simulink library "common_lib"  (R2021b)
settings: Solver=ode45  StartTime=0.0  StopTime=10.0  RelTol=1e-3
undefined symbols (not defined in the file or in its folder): ACCEL_PRE_MULT, C_C1GearNumbers, C_C1GearRatios, C_Calibration, C_DitherWaveform, C_GearOffset, C_GearRatioIn, C_GearRatioInverseOut, C_GearRatioOut, CLUTCH_INNER_LOOP_UPDATE_RATE, CONSTANT, DEGRADED_MODE_SIZE, Dem_EventStatusType, DiscIntNeverNeededParam, F_FAULT_ENUM, F_NOFAULT, F_OUTOFRANGE, F_RATELIMIT, FALSE, FMI14_SPECIAL_INSTRUCTIONS, FMI20_DATA_DRIFTED_HIGH, FMI21_DATA_DRIFTED_LOW, FMI29_RESERVED_FOR_SAE_ASSIGNMENT, FMI30_RESERVED_FOR_SAE_ASSIGNMENT, FMI31_CONDITION_EXISTS, FMI32_NO_FAULT, IC, k_accel, k_mean, LVDCU_OORH_FaultCntThd_C, MAX_UINT32, MEAN_PRE_MULT, NTriggers, QLTY_SIGNAL_FAILED, QLTY_SIGNAL_FULLY_FUNCTION, QLTY_SIGNAL_SUBSTITUTED_BY_1ST_CHOICE, QLTY_SIGNAL_SUBSTITUTED_BY_2ND_CHOICE, QLTY_SIGNAL_SUBSTITUTED_BY_3RD_CHOICE, QLTY_SIGNAL_SUBSTITUTED_BY_4TH_CHOICE, SAMPLE_TIME_100_mSec, SAMPLE_TIME_100_uSec, simin, T_TestPoint, TF_FALSE, TF_TRUE, TimeStep, TRUE, WORKSPACE_UPDATE_RATE, ZERO, Zero
libraries: $bdroot x120, simulink x27, simulink_extras x4, MBD_EPS_Local_Blockset x4
(part 2 of 10)

== system common_lib/Documentation ==
  note: Documentation
  EatonLogo : Subsystem
      mask Display: image('EatonLogo.jpg')
  LegalNoticeEaton : Subsystem  mask(LegalNotice){Company=Eaton Corporation}
      mask prompts: Company "Select Company"
      mask TypeOptions Company: Eaton Corporation | Eaton Cummins Automated Transmission Technologies
      mask Display:
      | corp = get_param(gcb,'Company');
      | disp(sprintf([...
      | 'Unpublished Work\n',...
      | 'Copyright %s %s.\n',...
      | 'Notice:\n',...
      | 'This document contains confidential information.\n',...
      | 'Disclosure of this information is conditioned upon the recipient''s agreement that\n',...
      | 'the use of the information shall be only for the purpose motivating the disclosure.\n',...
      | 'Any other use is strictly prohibited without the prior written consent.'],...
      | datestr(now,'yyyy'),corp))
  RequirementLinks : Subsystem  mask(ReqLink){}
      settings: OpenFcn=open_system([gcb '/DocBlock'])
      mask Display:
      | a = get_param([gcb '/DocBlock'],'UserData');
      | if isempty(a)
      |     disp('Double Click to Open');
      | else
      |     disp(sprintf('Requirements (REQ_####)\n%s',a.content));
      | end
  SubsystemPath : Subsystem  mask(SubSysPathInfo){}
      mask Display: disp(regexprep(get_param(gcb,'parent'),'/','>'))

== system common_lib/Fltrs ==
  note: Filters
  Fltr : Subsystem  RTWFcnName=FLTR  mask(CL Filter){TimeStep=[]}
      mask prompts: TimeStep "Time Step"
      mask help:
      | First Order Filter, y(n)= T/tau x(n) + (1 - T/tau) y(n-1)
      |
      | output = previous output + (input - previous output) * T/tau
      |
      | X(1) = input
      | X(2) = tau
      |
      | Y(1) = output
      |
      | Time step is entered via mask parameter.
      | NgEK, Inc.
      mask init:
      | %switch class(TimeStep)
      | %   case ('double')
      | %      IC = double(0.0);
      | %   case ('single')
      |        IC = single(0.0);
      | %   case ('int8')
      | %      IC = int8(0);
      | %   case ('int16')
      | %      IC = int16(0);
      | %   case ('int32')
      | %      IC = int32(0);
      | %end;
      | Ts = single(TimeStep);
      settings: RTWFcnNameOpts=User specified  RTWFileNameOpts=Use function name
      mask Help: web(which(['common_lib16.html']))
      mask Display:
      | patch([0.35 0.35 0.65 0.65], [0.4 0.6 0.6 0.4], [255/255 127/255 255/255])
      | disp('Filter')
      | port_label('input', 1, 'input')
      | port_label('input', 2, 'tau')
      | port_label('output', 1, 'output')
  Fltr_wR : Subsystem  mask(CL Filter wRO){TimeStep=[]}
      mask prompts: TimeStep "Time Step"
      mask help:
      | First Order Filter, y(n)= T/tau x(n) + (1 - T/tau) y(n-1)
      |
      | If      reset is true (1) then output=initial condition
      |    otherwise output = previous output + (input - previous output) * T/tau
      |
      | X(1) = input
      | X(2) = tau
      | X(3) = initial condition
      | X(4) = reset flag
      |
      | Y(1) = output
      |
      | Time step is entered via mask parameter.
      | NgEK, Inc.
      mask init: same as common_lib/Fltrs/Fltr
      mask Help: web(which(['common_lib18.html']))
      mask Display:
      | patch([0.4 0.4 0.6 0.6], [0.35 0.65 0.65 0.35], [255/255 127/255 255/255])
      | disp('Filter\nw R')
      | port_label('input', 1, 'input')
      | port_label('input', 2, 'tau')
      | port_label('input', 3, 'ic')
      | port_label('input', 4, 'reset?')
      | port_label('output', 1, 'output')
  Fltr_wRO : Subsystem  RTWFcnName=FLTRWRO  mask(CL Filter wRO){TimeStep=[]}
      mask prompts: TimeStep "Time Step"
      mask help:
      | First Order Filter, y(n)= T/tau x(n) + (1 - T/tau) y(n-1)
      |
      | If override is true (1) then output=override_value
      | If      reset is true (1) then output=input
      |    otherwise output = previous output + (input - previous output) * T/tau
      |
      | X(1) = input
      | X(2) = tau
      | X(3) = override value
      | X(4) = override flag
      | X(5) = reset flag
      |
      | Y(1) = output
      |
      | Time step is entered via mask parameter.
      | NgEK, Inc.
      mask init:
      | %switch class(TimeStep)
      | % case ('double')
      | %      IC = double(0.0);
      | %    case ('single')
      |        IC = single(0.0);
      | %    case ('int8')
      | %         IC = int8(0);
      | %    case ('int16')
      | %      IC = int16(0);
      | %   case ('int32')
      | %        IC = int32(0);
      | %end;
      | Ts = single(TimeStep);
      settings: RTWFcnNameOpts=User specified  RTWFileNameOpts=Use function name
      mask Help: web(which(['common_lib17.html']))
      mask Display:
      | patch([0.4 0.4 0.6 0.6], [0.35 0.65 0.65 0.35], [255/255 127/255 255/255])
      | disp('Filter\nw RO')
      | port_label('input', 1, 'input')
      | port_label('input', 2, 'tau')
      | port_label('input', 3, 'override_value')
      | port_label('input', 4, 'override?')
      | port_label('input', 5, 'reset?')
      | port_label('output', 1, 'output')
  Fltr_wROExtInitCond : Subsystem  TreatAsAtomicUnit=on  RTWFcnName=FLTRWRO  mask(CL Filter wRO wIC){TimeStep=[]}
      mask prompts: TimeStep "Time Step"
      mask help:
      | First Order Filter, y(n)= T/tau x(n) + (1 - T/tau) y(n-1)
      |
      | If override is true (1) then output=override_value
      | If      reset is true (1) then output=input
      |    otherwise output = previous output + (input - previous output) * T/tau
      |
      | X(1) = input
      | X(2) = tau
      | X(3) = inititial condition
      | X(4) = reset
      | X(5) = override TO
      | X(6) = override value TC
      | Y(1) = output
      mask init:
      | %switch class(TimeStep)
      | % case ('double')
      | %      IC = double(0.0);
      | %    case ('single')
      | %       IC = single(0.0);
      | %    case ('int8')
      | %         IC = int8(0);
      | %    case ('int16')
      | %      IC = int16(0);
      | %   case ('int32')
      | %        IC = int32(0);
      | %end;
      | %task_rate = single(taskrate_input);
      | Ts = single(TimeStep);
      settings: RTWFcnNameOpts=User specified  RTWFileNameOpts=Use function name
      mask Help: web(which(['common_lib17.html']))
      mask Display:
      | patch([0.2 0.2 0.8 0.8], [0.35 0.65 0.65 0.35], [255/255 127/255 255/255])
      | disp('Filter\n w ROExtInitCond')
      | port_label('input', 1, 'input')
      | port_label('input', 2, 'tau')
      | port_label('input', 3, 'ic')
      | port_label('input', 4, 'reset?')
      | port_label('input', 5, 'override?')
      | port_label('input', 6, 'override_value')
      | port_label('output',1, 'output')
  Int16FIR : Subsystem  mask(FIRInt16){N=50, Ts=0.01}
      mask prompts: N "Half Window Size (samples)"; Ts "Time Step"
      mask help:
      | Highly optimized FIR filter designed to calculated mean and least squares fit slope.
      |
      | For best results scale the input to use the whole range of int16, but note acceleration can saturate.  The buffer initializes to zero.
      |
      | Termination of an output will eliminate relevant code to calculate that output.
      mask init:
      | [k_mean, MEAN_PRE_MULT, k_accel, ACCEL_PRE_MULT] = FixedPointFIRInit(N,Ts);
      mask Display:
      | patch([0.35 0.35 0.65 0.65], [0.4 0.6 0.6 0.4], [255/255 127/255 255/255])
      | disp('Int16 FIR')
      | port_label('input', 1, 'u')
      | port_label('output', 1, 'mean')
      | port_label('output', 2, 'accel')
  Inv_Fltr : Subsystem  mask(CL Inverse Filter){TimeStep=[]}
      mask prompts: TimeStep "Time Step"
      mask help:
      | Inverse First Order Filter
      | u(k) = y(k-1) + tau/TimeStep*(y(k) - y(k-1))
      |
      | X(1) = input
      | X(2) = tau
      |
      | Y(1) = output
      |
      | Time step is entered via mask parameter.
      | NgEK, Inc.
      mask init:
      | %switch class(TimeStep)
      | %   case ('double')
      | %      Zero = double(0.0);
      | %   case ('single')
      |        Zero = single(0.0);
      | %   case ('int8')
      | %      Zero = int8(0);
      | %   case ('int16')
      | %      Zero = int16(0);
      | %   case ('int32')
      | %      Zero = int32(0);
      | %end;
      mask Help: web(which(['common_lib47.html']))
      mask Display:
      | patch([0.35 0.35 0.65 0.65], [0.3 0.7 0.7 0.3], [255/255 127/255 255/255])
      | disp('Inverse\nFilter')
      | port_label('input', 1, 'input')
      | port_label('input', 2, 'tau')
      | port_label('output', 1, 'output')
  Inv_RpdFltr : Subsystem  mask(CL Inverse Rapid Filtering){DType=Single}
      mask prompts: DType "Data Type"
      mask help:
      | Inverse of the Rapid Filter.  u(k) = y(k-1) + (y(k) - y(k-1))/fc
      |
      | X(1) = input
      | X(2) = filter constant
      |
      | Y(1) = output
      | NgEK, Inc.
      mask init:
      | switch class(TimeStep)
      |     case ('double')
      |         Zero = double(0.0);
      |     case ('single')
      |         Zero = single(0.0);
      |     case ('int8')
      |         Zero = int8(0);
      |     case ('int16')
      |         Zero = int16(0);
      |     case ('int32')
      |         Zero = int32(0);
      | end;
      mask Help: web(which(['common_lib48.html']))
      mask TypeOptions DType: Double | Single | Int8 | Int16 | Int32
      mask Display:
      | patch([0.30 0.30 0.70 0.70], [0.25 0.75 0.75 0.25], [255/255 127/255 255/255])
      | disp('Inverse\nRapid\nFiltering')
      | port_label('input', 1, 'input')
      | port_label('input', 2, 'fltr_cnst')
      | port_label('output', 1, 'output')
  Lookup_wFltr : Subsystem  mask(CL Filter wRO wIC wLut){TimeStep=[], Mode=Linear Interpolation}
      mask prompts: TimeStep "Time Step"; Mode "Interpolation Mode"
      mask help:
      | This block combines a 2D Table lookup with explicit axis inputs with a First Order Filter.
      |
      | First Order Filter, y(n)= T/tau x(n) + (1 - T/tau) y(n-1)
      |
      | If override is true (1) then output=override_value
      | If reset is true (1) then output=lookup_table_interpolation
      |    otherwise output = previous output + (lookup_table_interpolation - previous output) * T/tau
      |
      | X(1) = Independent variable
      | X(2) = X axis vector
      | X(3) = Y axis vector
      | X(4) = Override TO
      | X(5) = Override value TC
      | X(6) = Filter enable
      | X(7) = Filter tau
      | X(8) = Filter initial condition
      | Y(1) = Output
      |
      | Interpolation mode is selected via the mask:
      |
      | Ceiling Interpolation: rounds up in the positive direction
      | Floor Interpolation: rounds down in the negative direction
      | Nearest (Neighbor) Interpolation: rounds to the closest representable number
      | Linear Interpolation: Interpolates data by assuming data varies linearly between points
      mask init: same as common_lib/Fltrs/Fltr_wROExtInitCond
      mask TypeOptions Mode: Linear Interpolation | Nearest Neighbor | Floor | Ceiling
      mask Display:
      | patch([0.30 0.30 0.70 0.70], [0.45 0.55 0.55 0.45], [255/255 127/255 255/255])
      | disp('Lookup_wFltr')
      | port_label('input', 1, 'input')
      | port_label('input', 2, 'x-axis vector')
      | port_label('input', 3, 'y-axis vector' )
      | port_label('input', 4, 'override?')
      | port_label('input', 5, 'override_value')
      | port_label('input', 6, 'filter_enable?')
      | port_label('input', 7, 'tau')
      | port_label('input', 8, 'ic')
      | port_label('output', 1, 'output')
  Rpd_Fltr : Subsystem  mask(CL Rapid Filter){DType=Single}
      mask prompts: DType "Data Type"
      mask help:
      | Rapid 1st Order Filter, y(k)=x(k) + Fc*( Y(k-1) - X(k) )
      |
      | X(1) = input
      | X(2) = filter constant
      |
      | Y(1) = output
      | NgEK, Inc.
      mask init:
      | switch DType
      |    case (1)
      |        IC = double(0.0);
      |   case (2)
      |        IC = single(0.0);
      |    case (3)
      |          IC = int8(0);
      |     case (4)
      |          IC = int16(0);
      |    case (5)
      |        IC = int32(0);
      | end;
      mask Help: web(which(['common_lib19.html']))
      mask TypeOptions DType: Double | Single | Int8 | Int16 | Int32
      mask Display:
      | patch([0.35 0.35 0.65 0.65], [0.35 0.65 0.65 0.35], [255/255 127/255 255/255])
      | disp('Rapid\nFilter')
      | port_label('input', 1, 'input')
      | port_label('input', 2, 'fltr_cnst')
      | port_label('output', 1, 'output')
  Scaling_wFltr : Subsystem  mask(CL Filter wRO wIC wScl){TimeStep=[]}
      mask prompts: TimeStep "Time Step"
      mask help:
      | This block adds sclaing to scale the raw input signal. The signal is then filtered using first order filter.
      |
      | First Order Filter, y(n)= T/tau x(n) + (1 - T/tau) y(n-1)
      |
      | If override is true (1) then output=override_value
      | If reset is true (1) then output=input*resolution+offset
      |    otherwise output = previous output + ((input*resolution+offset) - previous output) * T/tau
      |
      | X(1) = input
      | X(2) = resolution
      | X(3) = offset
      | X(4) = override TO
      | X(5) = override value TC
      | X(6) = filter enable
      | X(7) = filter tau
      | X(8) = filter initial condition
      | Y(1) = output
      mask init: same as common_lib/Fltrs/Fltr_wROExtInitCond
      mask Display:
      | patch([0.30 0.30 0.70 0.70], [0.45 0.55 0.55 0.45], [255/255 127/255 255/255])
      | disp('Scaling_wFltr')
      | port_label('input', 1, 'input')
      | port_label('input', 2, 'res')
      | port_label('input', 3, 'offset' )
      | port_label('input', 4, 'override?')
      | port_label('input', 5, 'override_value')
      | port_label('input', 6, 'filter_enable?')
      | port_label('input', 7, 'tau')
      | port_label('input', 8, 'ic')
      | port_label('output', 1, 'output')

== system common_lib/Fuzzy ==
  note: Fuzzy Controller Design
  Demux : Demux  Outputs=2
  Fuzzy Implication : Subsystem  mask(CL Fuzzy Implication){from=ShiftPoint, value=HighUpshiftPoint}
      mask prompts: from "Result Bus Goto Tag"
      mask help:
      | The fuzzy implication is the final result of a decision tree branch.
      |
      | The value parameter of this block selects from the Result Bus the particular value that the output should take on when the associated branch is true.
      |
      | It is ok and likely to have multiple branches that result in the same value.  Adding all the result branches together will give a weight sum of the result.
      mask init:
      | set_param([gcb '/From'],'GotoTag',get_param(gcb,'from'));
      | set_param([gcb '/Select'],'OutputSignals',get_param(gcb,'value'))
      mask Display:
      | patch([0.25 0.25 0.75 0.75], [0.25 0.75 0.75 0.25], [255/255 127/255 255/255])
      | port_label('input',1,'THEN');
      | disp([get_param(gcb,'from') ' is\n' get_param(gcb,'value')])
  Fuzzy Intersection : Subsystem  mask(CL Fuzzy Decision){from=DataBus, signal=Demand, value=value, dispStr=Demand is\nvalue}
      mask prompts: from "Data Bus Goto Tag"; signal "Signal Name"; value "Value(s) (Comma seperated list of named values)"
      mask help:
      | The Fuzzy Decision block serves as the fuzzy AND operator.
      |
      | Input - Truth of previous statements.
      | TRUE Output - Incoming truth AND truth of selected signal values(s).
      | FALSE Output - Incoming truth AND falseness of selected signal values(s).
      |
      | TRUE Output + FALSE Output = Input
      mask init:
      | fromDlg = get_param(gcb,'from');
      | fromBlk = get_param([gcb '/From'],'GotoTag');
      | if ~strcmp(fromDlg,fromBlk)
      |    set_param([gcb '/From'],'GotoTag',get_param(gcb,'from'));
      | end
      | 
      | remain = strtrim(get_param(gcb,'value'));
      | first = true;
      | output = '';
      | sig = get_param(gcb,'signal');
      | dstr = [sig ' is\n'];
      | while any(remain)
      |     [str, remain] = strtok(remain,{',',' '});
      |     if first
      |         output = [sig '.' str];
      |         dstr = [dstr str];
      |     else
      |         output = [output ',' sig '.' str];
      |         dstr = [dstr '\nOR ' str];
      |     end
      |     first = false;
      | end
      | 
      | if ~strcmp(get_param(gcb,'dispStr'),dstr) || ...
      |    ~strcmp(get_param([gcb '/Select'],'OutputSignals'),output)
      |    set_param(gcb,'dispStr',dstr);
      | 
      |    %Delete old lines
      |    sel = get_param([gcb '/Select'],'PortHandles');
      |    n = length(sel.Outport);
      |    for i = 1:n
      |        line = get(sel.Outport(i),'Line');
      |        if line>0
      |            delete_line(line);
      |        end
      |    end
      | 
      |    %Set the new outputs
      |    set_param([gcb '/Select'],'OutputSignals',output)
      | 
      |    %Add new lines
      |    sel = get_param([gcb '/Select'],'PortHandles');
      |    n = length(sel.Outport);
      |    set_param([gcb '/OR'],'Inputs',char(ones(1,n)*'+'));
      |    for i = 1:n
      |        istr = num2str(i);
      |        add_line(gcb,['Select/' istr],['OR/' istr]);
      |    end
      | end
      mask Help:
      | The Fuzzy Decision block serves as the fuzzy AND operator.  The TRUE output
      | is the truth of the input AND truth of the selected signal value(s).  The
      | FALSE output is truth of the input but falseness of the selected signal
      | value(s).  Thus the sum of TRUE and FALSE output will equal the truth of
      | the input.
      | 
      | Use this block as nodes in a binary decision tree.  The root node should
      | always have an input truth of 1.0, the sum of all branches.  At the end of
      | each branch should be a Fuzzy THEN statement followed by a summation of all
      | THEN statements.
      mask Callback value:
      | if isempty(strtrim(get_param(gcb,'value')))
      |     set_param(gcb,'value','value');
      | end
      mask Display:
      | patch([0.25 0.25 0.75 0.75], [0.25 0.75 0.75 0.25], [255/255 127/255 255/255])
      | port_label('input',1,'IF');
      | port_label('output',1,'THEN');
      | port_label('output',2,'ELSE');
      | disp(get_param(gcb,'dispStr'))
  Fuzzy Membership Function : Subsystem  mask(CL Fuzzy Membership){}
      mask help:
      | This fuzzy membership function uses triangular functions centered at the breakpoints defined by the second input.  A ramp function is used for the first and last break point.
      |
      | This membership function enforces the property of mutual exclusivity.  The sum of all memberships equals 1.0 for the range of the input.
      |
      | The breakpoints must be in increasing order and be unique.  If not, order and uniqueness will be enforced by shifting breakpoints above the previously listed value in an iterative fasion.
      |
      | First Input - Input signal
      | Second Input - Breakpoint list
      mask Display:
      | patch([0.22 0.22 0.8 0.8], [0.3 0.68 0.68 0.3], [255/255 127/255 255/255])
      | plot([0.0 0.4 0.4],[0.8 0.8 0.7]);
      | text(0.15,0.65,'1');
      | plot([0.2 0.3 0.5 0.8],[0.7 0.7 0.3 0.3]);
      | plot([0.3 0.5 0.7],[0.3 0.7 0.3]);
      | text(0.15,0.35,'0');
      | plot([0.2 0.5 0.7 0.8],[0.3 0.3 0.7 0.7]);
      | 
      | 
      | plot([0.0 0.3 0.3 0.3 0.5 0.5 0.5 0.7 0.7],[0.2 0.2 0.25 0.2 0.2 0.25 0.2 0.2 0.25])
  Fuzzy Union : Sum  Inputs=|++
  Goto Tag Visibility : GotoTagVisibility  GotoTag=DataBus
  Goto Tag Visibility1 : GotoTagVisibility  GotoTag=ResultBus
  Truth : Constant  Value=single(1.0)  SampleTime=-1

== system common_lib/Gear Ratios ==
  note: Gear Ratios
  FindGearNumberByRatio : Subsystem  mask{RatioToGearIn=C_C1GearRatios, RatioToGearOut=C_C1GearNumbers, GearToRatioIn=C_GearRatioIn, GearToRatioOut=C_GearRatioOut, ConfirmTime=single(0), TimeStep=0.001}
      mask prompts: RatioToGearIn "RatioToGearIn (single)"; RatioToGearOut "RatioToGearOut (single)"; GearToRatioIn "GearToRatioIn (single)"; GearToRatioOut "GearToRatioOut (single)"; ConfirmTime "Speeed Confirmation Time (single)"; TimeStep "Time Step (double)"
      mask help:
      | This block outputs the GearNumber closest to the ratio appearing at the
      | input.  The block requires monotonically increasing tables.  i.e. the
      | RatioToGearIn and GearToRatioIn values must be increasing.
      |
      | The block works for both forward and reverse ratios.  (Positive and negative
      | speed and ratio).
      |
      | GearNumber - The gear number of the determined ratio.  Set to single(0) if
      | ratio does not match an available ratio.
      |
      | OutputValid - True if the ratio matches for ConfirmTime and above MinSpeed.
      |
      | SpeedAboveMin - True if speed is above MinSpeed.
      |
      | Ratio = ClutchSpeed/OutputSpeed
  GearNumberToRatio : Subsystem
      mask Display:
      | patch([0.3 0.3 0.7 0.7], [0.4 0.6 0.6 0.4], [255/255 127/255 255/255]);
      | disp('Gear Num\n to Ratio')
      | port_label('input',1,'gear_num')
      | port_label('output',1,'ratio')
      | port_label('output',2,'inv_ratio')

== system common_lib/IO ==
  note: IO Blocks
  Calibration with Pretty Print Value : Subsystem  mask(Calibratible Input){CalValue=C_Calibration, scaling=None}
      mask prompts: CalValue "Calibratible Name"
      mask help:
      | This block is simply a standard Simulink constant block w/ a custom wrapper to pretty-print the calibratible value on the mask.
      |
      | NgEK, Inc.
      mask init:
      | CalName = get_param(gcb,'CalValue');
      mask TypeOptions scaling: None | RPM | MPH
      mask Display:
      | fprintf([CalName ' = ' num2str(double(CalValue)*...
      |     (strcmp(get_param(gcb,'scaling'),'RPM')*30/pi+...
      |      strcmp(get_param(gcb,'scaling'),'MPH')*2.236936292+...
      |      strcmp(get_param(gcb,'scaling'),'None')*1.0)) ' '...
      |      char(strcmp(get_param(gcb,'scaling'),'RPM')*double('RPM')+...
      |           strcmp(get_param(gcb,'scaling'),'MPH')*double('MPH')+...
      |           strcmp(get_param(gcb,'scaling'),'None')*double(sprintf('   ')))])
  Calibration with Pretty Print Value1 : $bdroot/IO/Calibration with Pretty Print Value  CalValue=c_Calibration  scaling=None
  From Workspace w/Datatype : Subsystem  mask(From Workspace w/Datatype){st=0, var=simin, intdat=on, zerocross=off, extmode=Extrapolation}
      mask prompts: st "sample time"; var "data"; intdat "Interpolate data"; zerocross "Enable zero crossing detection"; extmode "Form output after final data value by:"
      mask help:
      | From worspace block with data type convertor at its output.
      |
      | NgEK, Inc.
      mask init:
      | dt = get_param(gcb,'st');
      | data = get_param(gcb,'var');
      | blk = [gcb '/From' sprintf('\n') 'Workspace'];
      | if intdat, mode = 'on'; else mode = 'off'; end
      | set_param(blk,'interpolate',mode)
      | if zerocross, mode = 'on'; else mode = 'off'; end
      | set_param(blk,'zerocross',mode)
      | switch extmode
      |     case 1
      |         mode = 'Extrapolation';
      |     case 2
      |         mode = 'Setting to zero';
      |     case 3
      |         mode = 'Hold final value';
      |     case 4
      |         mode = 'Cyclic repetition';
      | end
      | set_param(blk,'outputafterfinalvalue',mode)
      mask Help: Use just like the original from workspace block.
      mask TypeOptions extmode: Extrapolation | Setting to zero | Holding final value | Cyclic repetition
      mask Display: disp(data)
  Triangle : Subsystem  mask(CL Triangle){TimeStep=[]}
      mask prompts: TimeStep "Time Step"
      mask help:
      | Output a triangle signal of specified amplitude, offset and frequency.
      |
      | X(1) = amplitude
      | X(2) = frequency
      | X(3) = offset
      |
      | Y(1) = output
      |
      | Time step is entered via mask parameter.
      | NgEK, Inc.
      mask init:
      | h=[gcb '/Data Type Conversion'];
      | 
      | %switch class(TimeStep)
      | %   case ('double')
      | %      Zero        = double( 0.0);
      | %      ZeroZeroOne = double( 0.001);
      | %      One         = double( 1.0);
      | %      Two         = double( 2.0);
      | %      MinusOne    = double(-1.0);
      | %      set_param(h, 'DataType','double');
      | %      set_param([h '1'], 'DataType','double');
      | %   case ('single')
      |        Zero        = single( 0.0);
      |        ZeroZeroOne = single( 0.001);
      |        One         = single( 1.0);
      |        Two         = single( 2.0);
      |        MinusOne    = single(-1.0);
      |        set_param(h, 'DataType','single');
      |        set_param([h '1'], 'DataType','single');
      | %end;
      mask Help: web(which(['common_lib20.html']))
      mask Display:
      | patch([0.375 0.375 0.625 0.625], [0.35 0.65 0.65 0.35], [255/255 127/255 255/255])
      | plot([0.375 0.4375 .5 0.5625 0.625],[0.35 0.65 0.35 0.65 0.35]);
      | port_label('input', 1, 'amplitude')
      | port_label('input', 2, 'frequency')
      | port_label('input', 3, 'offset')
      | port_label('output', 1, 'output')

== system common_lib/Integrators ==
  note: Integrators
  ForwardEulerIntergrator : Subsystem  mask{IC=0, TSAMP=0}
      mask prompts: IC "Initial Condition"; TSAMP "Sample Time"
      mask Display:
      | patch([0.35 0.35 0.65 0.65], [0.3 0.7 0.7 0.3], [255/255 127/255 255/255])
      | disp('Forward Euler\nIntegral')
      | port_label('input',1,'dx')
      | port_label('input',2,'x0')
      | port_label('input',3,'reset')
      | port_label('output',1,'x')

== system common_lib/Misc ==
  note: Miscellaneous Computations
  ArcSine : Subsystem  mask(CL Trigonometric Function ArcSine){}
      mask help:
      | Simple trigonometric arcsine function.  The sine is the input and the angle is the output.
      |
      | This block is single precision.  The calculation used to determine arcsine is dervied from a Taylor Series approximation.  Note there are limitations with this approximation such as round off error.
      |
      | NgEK, Inc.
      mask Help: web(which(['common_lib51.html']))
      mask Display:
      | patch([0.30 0.30 0.70 0.70], [0.25 0.75 0.75 0.25], [255/255 127/255 255/255])
      | plot(linspace(-1,1,20)/6+0.5,(asin(linspace(-1,1,20)))/6.28+0.5)
  ClampAboveZero : Subsystem  mask(CL Clamp Above Zero){Tol=[]}
      mask prompts: Tol "Tolerance"
      mask help:
      | Clamps input above zero according to a calibratible tolerance.
      |
      | X(1) = input
      |
      | Y(1) = output
      | NgEK, Inc.
      settings: AttributesFormatString=tol=%<Tol>
      mask Help: web(which(['common_lib21.html']))
      mask Display:
      | patch([0.3 0.3 0.7 0.7], [0.35 0.65 0.65 0.35], [255/255 127/255 255/255])
      | 
      | plot([0 1],[0.5 0.5], [0.5 0.5],[0 1], [0 0.5 1], [0.55 0.55 1])
  ClampAroundZero : Subsystem  mask(CL Clamp Around Zero){Tol=[]}
      mask prompts: Tol "Tolerance"
      mask help:
      | Clamps input around zero according to a calibratible tolerance.
      |
      | X(1) = input
      |
      | Y(1) = output
      | NgEK, Inc
      mask init:
      | switch class(Tol)
      |   case ('double')
      |       One      = double(1.0);
      |        Zero     = double(0.0);
      |        MinusOne = double(-1.0);
      |  case ('single')
      |         One      = single(1.0);
      |        Zero     = single(0.0);
      |          MinusOne = single(-1.0);
      |  case ('int8')
      |         One      = int8(1.0);
      |          Zero     = int8(0.0);
      |          MinusOne = int8(-1.0);
      |     case ('int16')
      |        One      = int16(1.0);
      |         Zero     = int16(0.0);
      |         MinusOne = int16(-1.0);
      |   case ('int32')
      |         One      = int32(1.0);
      |         Zero     = int32(0.0);
      |         MinusOne = int32(-1.0);
      | end;
      settings: AttributesFormatString=tol=%<Tol>
      mask Help: web(which(['common_lib22.html']))
      mask Display:
      | patch([0.3 0.3 0.7 0.7], [0.35 0.65 0.65 0.35], [255/255 127/255 255/255])
      | 
      | plot([0 1],[0.5 0.5], [0.5 0.5],[0 1], [0 0.3 0.5 0.5 0.7 1], [0 0.3 0.3 0.7 0.7 1])
  Cosine : Subsystem  mask(CL Trigonometric Function Cosine){}
      mask help:
      | Simple trigonometric cosine function.  The angle is the input and the cosine angle is the output.
      |
      | This block is single precision.  The calculation used to determine cosine is dervied from a Taylor Series approximation.  Note there are limitations with this approximation such as round off error.
      |
      | NgEK, Inc.
      mask Help: web(which(['common_lib52.html']))
      mask Display:
      | patch([0.30 0.30 0.70 0.70], [0.25 0.75 0.75 0.25], [255/255 127/255 255/255])
      | plot(linspace(0,6.28,20)/16+0.3,(1+cos(linspace(0,6.28,20)))/4+0.25)
  Count Edges : Subsystem  mask(CL Count Edges){}
      mask help:
      | Generic counter
      |
      | Counts the number of edges from FALSE to TRUE.  Includes reset input to set the count back to zero.
      mask Help: web(which(['common_lib54.html']))
      mask Display:
      | patch([0.30 0.30 0.70 0.70], [0.25 0.75 0.75 0.25], [255/255 127/255 255/255])
      | disp('Count Edges')
  Count to X : Subsystem  mask(CL Count To X){X=, edge=FALSE to TRUE}
      mask prompts: X "Divide by count"; edge "Count edge"
      mask help:
      | Generic count to X
      | Outputs a TRUE after X edges.
      |
      | Edge polarity and X are set by mask.
      | NgEK, Inc.
      mask init:
      | h_input      = [gcb '/Input'];
      | h_dinput    = [gcb '/DelayedInput'];
      | 
      | switch get_param(gcb,'edge')
      |    case 'FALSE to TRUE'
      |       set_param(h_input,  'Operator','AND');
      |         set_param(h_dinput, 'Operator','NAND');
      |  otherwise
      |      set_param(h_input,  'Operator','NAND');
      |         set_param(h_dinput, 'Operator','AND');
      | end
      mask Help: web(which(['common_lib26.html']))
      mask TypeOptions edge: FALSE to TRUE | TRUE to FALSE
      mask Display:
      | patch([0.1 0.1 0.9 0.9], [0.2 0.8 0.8 0.2], [255/255 127/255 255/255])
      | disp([...
      |        'Count to ' get_param(gcb,'X') '\n'...
      |        get_param(gcb,'edge')...
      |   ])
      | port_label('input',1,'in');
      | port_label('input',2,'reset?');
      | port_label('output',1,'out');
  Counter : Subsystem  mask(CL Counter){IC=[]}
      mask prompts: IC "Initial condition"
      mask help:
      | Generic counter block.
      | Counts up by up_val when count_up? is true
      | Counts down by down_val when count_down? is true.
      | Block can be used as a timer if increment value is set to the frame rate.
      |
      | X(1) = increment value
      | X(2) = count up flag
      | X(3) = decrement value
      | X(4) = count down flag
      | X(5) = max counter value
      | X(6) = min counter value
      | X(7) = reset
      |
      | Y(1) = output
      |
      | Initial condition is entered via mask.
      | NgEK, Inc.
      mask init:
      | switch class(IC)
      |    case ('double')
      |         Zero     = double(0.0);
      |   case ('single')
      |        Zero     = single(0.0);
      |   case ('int8')
      |       Zero     = int8(0.0);
      |     case ('uint16')
      |        Zero     = uint16(0.0);
      |  case ('uint32')
      |         Zero     = uint32(0.0);
      |     case ('int16')
      |         Zero     = int16(0.0);
      |    case ('int32')
      |         Zero     = int32(0.0);
      | end;
      mask Help: web(which(['common_lib23.html']))
      mask Display:
      | patch([0.4 0.4 0.6 0.6], [0.4 0.6 0.6 0.4], [255/255 127/255 255/255])
      | disp('Counter')
      | port_label('input', 1, 'up_val')
      | port_label('input', 2, 'count_up?')
      | port_label('input', 3, 'down_val')
      | port_label('input', 4, 'count_down?')
      | port_label('input', 5, 'max_count')
      | port_label('input', 6, 'min_count')
      | port_label('input', 7, 'reset?')
      | port_label('output', 1, 'output')
  Divide by X : Subsystem  mask(CL Divide By X){X=[]}
      mask prompts: X "Divide by count"
      mask help:
      | Generic divide by X
      | Outputs a true every X iterations.
      |
      | trigger? input forces output true
      |
      | Divide by X  is entered via mask.
      | NgEK, Inc.
      mask Help: web(which(['common_lib25.html']))
      mask Display:
      | patch([0.3 0.3 0.7 0.7], [0.4 0.6 0.6 0.4], [255/255 127/255 255/255])
      | disp(['Divide by ' num2str(X)])
      | port_label('input', 1, 'trigger?')
      | port_label('output', 1, 'output')
  EatonLogo : Subsystem
      mask Display: image(imread('EatonLogo.jpg'));
  EdgeTriggered Pulse : Subsystem  RTWFcnName=ETP  mask(CL Edge Triggered Pulse){Edge=TRUE to FALSE, Width=[], Pulse=TRUE, TimeStep=[], Init=0}
      mask prompts: Edge "Edge Detection"; Width "Pulse Width (seconds)"; Pulse "Pulse Value (boolean)"; TimeStep "Time Step"; Init "N/A"
      mask help:
      | Upon detection of an edge on the input (TRUE to FALSE or FALSE to TRUE)
      | output a pulse (TRUE or FALSE).
      |
      | Edge detect, pulse value, pulse width and update rate (the last two are SINGLE type) are entered via the mask.
      | NgEK, Inc.
      mask init:
      | set_param([gcb '/ETP'],'Edge',get_param(gcb,'Edge'));
      | set_param([gcb '/ETP'],'Pulse',get_param(gcb,'Pulse'));
      | set_param([gcb '/ETP'],'TimeStep',get_param(gcb,'TimeStep'));
      settings: RTWFcnNameOpts=User specified  RTWFileNameOpts=Use function name
      mask Help: web(which(['common_lib28.html']))
      mask TypeOptions Edge: FALSE to TRUE | TRUE to FALSE
      mask TypeOptions Pulse: TRUE | FALSE
      mask Display:
      | patch([0.02 0.02 0.98 0.98], [0.1 0.9 0.9 0.1], [255/255 127/255 255/255]);
      | disp([...
      |       'Edge= ' get_param(gcb,'edge') '\n'...
      |       'Width= ' get_param(gcb,'width') '\n'...
      |       'Pulse Value= ' get_param(gcb,'pulse')...
      |  ]);
  EdgeTriggered Pulse w time : Subsystem  RTWFcnName=ETPWT  mask(CL Edge Triggered Pulse w Time){Edge=TRUE to FALSE, Pulse=FALSE, TimeStep=[], Init=0}
      mask prompts: Edge "Edge Detection"; Pulse "Pulse Value (boolean)"; TimeStep "Time Step"; Init "N/A"
      mask help:
      | Upon detection of an edge on the input (TRUE to FALSE or FALSE to TRUE)
      | output a pulse (TRUE or FALSE).
      |
      | Edge detect, pulse value, pulse width and update rate (the last two are SINGLE type)
      | are entered via the mask.
      | NgEK, Inc.
      mask init:
      | switch get_param(gcb,'Edge')
      |     case 'FALSE to TRUE'
      |        TRIGGER=false;
      |    otherwise
      |        TRIGGER=true;
      | end
      | 
      | switch get_param(gcb,'Pulse')
      |    case 'FALSE'
      |       OUTPUT = false;
      |    otherwise
      |       OUTPUT = true;
      | end
      | Ts = single(TimeStep);
      | Ts_half = Ts/single(2.0);
      settings: RTWSystemCode=Inline  RTWFcnNameOpts=User specified  RTWFileNameOpts=Use function name
      mask Help: web(which(['common_lib29.html']))
      mask TypeOptions Edge: FALSE to TRUE | TRUE to FALSE
      mask TypeOptions Pulse: TRUE | FALSE
      mask Display:
      | patch([0.02 0.02 0.98 0.98], [0.1 0.9 0.9 0.1], [255/255 127/255 255/255]);
      | disp([...
      |       'Edge= ' get_param(gcb,'edge') '\n'...
      |       'Pulse Value= ' get_param(gcb,'pulse')...
      |     ]);
  GreenLeaf_Globe : Subsystem
      mask Display: image(imread('greenleaf_globe.png'));
  Hold : Subsystem  TreatAsAtomicUnit=on
      settings: RTWSystemCode=Inline
      mask Display:
      | patch([0.25 0.25 0.75 0.75], [0.05 0.3 0.3 0.05], [255/255 127/255 255/255])
      | disp('\n\nHold');
  Latch : Subsystem  mask(CL Latch){IC=[]}
      mask prompts: IC "Initial Condition"
      mask help:
      | Input is latched until reset is true
      |
      | X(1) = input
      | X(2) = reset
      |
      | Y(1) = output
      |
      | Initial condition is entered via mask.
      | NgEK, Inc.
      mask Help: web(which(['common_lib24.html']))
      mask Display:
      | patch([0.35 0.35 0.65 0.65], [0.3 0.65 0.65 0.3], [255/255 127/255 255/255])
      | disp('Latch')
      | port_label('input', 1, 'input')
      | port_label('input', 2, 'reset?')
      | port_label('output', 1, 'output')
  ModelVersion : Subsystem  mask{MdlVer=0}
      mask prompts: MdlVer "Model Version"
      mask init:
      | % Use the simulink model verison
      | mdlName = get_param(bdroot,'name'); 
      | % mdlVersionStr = get_param(bdroot,'Modelversion');
      | % mdlVersion = single(str2num(mdlVersionStr));
      | % mdlVersionSignal =[strrep(mdlName,'SWC_','') '_SwcVer'];
      | 
      | mdlVersion = uint8(MdlVer);
      | mdlVersionSignal =[strrep(mdlName,'SWC_','') '_SwcVer'];
      | 
      | %Set the signal name to match the SwC
      | p = get_param([gcb '/mdlVersionBlock'],'PortHandles');
      | l = get_param(p.Outport,'Line');
      | set_param(l,'Name',mdlVersionSignal);
      | set_param(p.Outport,'MustResolveToSignalObject','on');
      | 
      | %Open the data dictionary
      | try
      |     myDictionaryObj = ...
      |     Simulink.data.dictionary.open([mdlName '.sldd']);
      |     dDataSectObj = getSection(myDictionaryObj,'Design Data');
      | 
      |     %Check if the signal object is present
      |     %foundEntries = find(dDataSectObj,'Name',mdlVersionSignal,'-class','Simulink.Signal');
      | 
      |     if ~exist(dDataSectObj,mdlVersionSignal)
      |         entryDiction = addEntry(dDataSectObj,mdlVersionSignal,Simulink.Signal);
      |         entrySub = Simulink.Signal;
      |         entrySub.DataType = 'uint8';
      |         entrySub.Min = 0;
      |         entrySub.CoderInfo.StorageClass = 'ExportedGlobal'
      |         setValue(entryDiction,entrySub);
      |         saveChanges(myDictionaryObj);
      |     end        
      |     close(myDictionaryObj); 
      |     
      | catch
      |     
      | end
      mask DialogControl DescTextVar Prompt: This model adds correct signal object to display the correct model version
      mask Display: disp('Model Version')
  Sine : Subsystem  mask(CL Trigonometric Function Sine){}
      mask help:
      | Simple trigonometric sine function.  The angle is the input and the sine angle is the output.
      |
      | This block is single precision.  The calculation used to determine sine is dervied from a Taylor Series approximation.  Note there are limitations with this approximation such as round off error.
      |
      | NgEK, Inc.
      mask Help: web(which(['common_lib51.html']))
      mask Display:
      | patch([0.30 0.30 0.70 0.70], [0.25 0.75 0.75 0.25], [255/255 127/255 255/255])
      | plot(linspace(0,6.28,20)/16+0.3,(1+sin(linspace(0,6.28,20)))/4+0.25)
  Tangent : Subsystem  mask(CL Trigonometric Function Sine){}
      mask help:
      | Simple trigonometric tangent function.  The angle is the input and the tan angle is the output.
      |
      | This block is single precision.  The calculation used to determine tangent is dervied from a Taylor Series approximation.  Note there are limitations with this approximation such as round off error.
      |
      | NgEK, Inc.
      mask Help: web(which(['common_lib53.html']))
      mask Display:
      | patch([0.30 0.30 0.70 0.70], [0.25 0.75 0.75 0.25], [255/255 127/255 255/255])
      | plot(linspace(0,6.28,20)/16+0.3,(1+tan(linspace(0,6.28,20)))/10+0.25)
  Timeout Detection : Subsystem  RTWFcnName=TIMEOUT  mask(CL Timeout){Timeout=, TimeStep=}
      mask prompts: Timeout "Timeout  (seconds)"; TimeStep "Time Step"
      mask help:
      | Timeout detection monitors the input
      | and signals a TRUE if the input is unchanging
      | for longer than the timeout interval.
      |
      | Update Rate and Timeout are entered via the mask.
      | NgEK, Inc.
      mask init:
      | % switch class(Timeout)
      | %   case ('double')
      | %        Tol      = double(TimeStep)/2.0;
      | %       Zero     = double(0.0);
      | %   case ('single')
      | %         Tol      = single(double(TimeStep)/2.0);
      | %         Zero     = single(0.0);
      | %    case ('int8')
      | %       Tol      = int8(double(TimeStep)/2.0);
      | %          Zero     = int8(0.0);
      | %     case ('int16')
      | %         Tol      = int16(double(TimeStep)/2.0);        
      | %       Zero     = int16(0.0);
      | %    case ('int32')
      | %          Tol      = int32(double(TimeStep)/2.0);       
      | %        Zero     = int32(0.0);
      | % end;
      | 
      | Ts = single(TimeStep);
      | Tol = Ts/single(2.0);
      | Zero = single(0.0);
      settings: RTWFcnNameOpts=User specified  RTWFileNameOpts=Use function name
      mask Help: web(which(['common_lib27.html']))
      mask Display:
      | patch([0.05 0.05 0.95 0.95], [0.15 0.85 0.85 0.15], [255/255 127/255 255/255]);
      | disp(['Timeout = \n' get_param(gcb,'Timeout')]);
  Timeout with time : Subsystem  RTWFcnName=TIMEOUT  mask(CL Timeout){TimeStep=[]}
      mask prompts: TimeStep "Time Step"
      mask help:
      | Timeout detection monitors the input
      | and signals a TRUE if the input is unchanging
      | for longer than the timeout interval.
      |
      | Update Rate and Timeout are entered via the mask.
      | NgEK, Inc.
      mask init: same as common_lib/Misc/Timeout Detection
      settings: RTWFcnNameOpts=User specified  RTWFileNameOpts=Use function name
      mask Help: web(which(['common_lib27.html']))
      mask Display:
      | patch([0.05 0.05 0.95 0.95], [0.15 0.85 0.85 0.15], [255/255 127/255 255/255]);
      | disp(['Timeout = \n Input Port 2' ]);
  Value Latch1 : Subsystem  mask(CL Latch){IC=, HoldTime=0, TimeStep=0}
      mask prompts: IC "Initial Condition"; HoldTime "Hold Time"; TimeStep "Time Step"
      mask help:
      | Input is latched until reset is true
      |
      | X(1) = input
      | X(2) = reset
      |
      | Y(1) = output
      |
      | Initial condition is entered via mask.
      | NgEK, Inc.
      mask Help: web(which(['common_lib24.html']))
      mask Display:
      | patch([0.35 0.35 0.65 0.65], [0.3 0.65 0.65 0.3], [255/255 127/255 255/255])
      | disp('Latch')
      | port_label('input', 1, 'input')
      | port_label('output', 1, 'output')

== system common_lib/OS ==
  note: These components are atomic elements used by the
      | schedule_morph script to build scheduler blocks
  note: OS Components
  Scheduler : Subsystem  mask(CL Scheduler){Number=5, DType=Fcn_Call, Style=Trigger all tasks each frame, State=off}
      mask prompts: Number "Number of Tasks to Trigger"; DType "Type of Trigger"; Style "Schedule Style"; State "Display Scheduler State"
      mask help:
      | Simulink-based task scheduler capable of generating  boolean or fcn_call triggers.  Tasks may be staggered so that one is executed each frame in a round-robin fashion or all tasks may be triggered in sequence in a single frame.
      |
      | Boolean output for all tasks triggering in a frame is not implemented yet.
      |
      | NgEK, Inc.
      mask init:
      | NTriggers=int8(max([Number 1]));
      | TRUE = boolean(1);
      | FALSE = boolean(0);
      | schedule_morph;
      settings: RTWSystemCode=Nonreusable function  RTWFcnNameOpts=Use subsystem name  RTWFileNameOpts=Use subsystem name
      mask Help: web(which(['common_lib30.html']))
      mask TypeOptions DType: Boolean | Fcn_Call
      mask TypeOptions Style: Trigger one task per frame | Trigger all tasks each frame
      mask Display:
      | patch([0.3 0.3 0.7 0.7], [0.35 0.65 0.65 0.35], [255/255 127/255 255/255])
      | disp('Scheduler');
      | 
      | port_label('output',1,'Task 1');
      | port_label('output',2,'Task 2');
      | port_label('output',3,'Task 3');
      | port_label('output',4,'Task 4');
      | port_label('output',5,'Task 5');
  Scheduler with Init : Subsystem  mask(CL Scheduler with Init){Number=2}
      mask prompts: Number "Number of Tasks to Trigger"
      mask help:
      | Simulink-based task scheduler capable of generating  fcn_call triggers.  Tasks are triggered in sequence in a single frame.  The task wired to the "Init" port is only executed in the first frame.
      |
      | NgEK, Inc.
      mask init:
      | NTriggers=int8(max([Number 1]));
      | TRUE = boolean(1);
      | FALSE = boolean(0);
      | schedule_morph2;
      settings: RTWSystemCode=Nonreusable function  RTWFcnNameOpts=Use subsystem name  RTWFileNameOpts=Use subsystem name
      mask Help: web(which(['common_lib55.html']))
      mask Display:
      | patch([0.3 0.3 0.7 0.7], [0.35 0.65 0.65 0.35], [255/255 127/255 255/255])
      | disp('Scheduler\nwith Init');
      | 
      | port_label('output',1,'Init');
      | port_label('output',2,'Task 1');
      | port_label('output',3,'Task 2');
  fcn_call generator : Subsystem  TreatAsAtomicUnit=on
  schedule counter : Subsystem
  sequence generator : Subsystem  TreatAsAtomicUnit=on
